simulink model "img_processing"  (R2019b)
settings: Solver=VariableStepAuto  StartTime=0.0  StopTime=10.0  RelTol=1e-3
undefined symbols (not defined in the file or in its folder): none
libraries: imaqlib x1
settings Model: Creator=James  LastModifiedBy=James

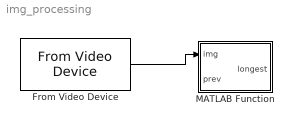
== system img_processing ==
  From Video Device : imaqlib/From Video Device  DeviceMenu=(none)  Device=(none)  ObjConstructor=(none)  VideoFormatMenu=(none)  VideoFormat=(none)  VideoSource=none  ROIPosition=(none)  EnableHWTrigger=off  TriggerConfiguration=none/none  SampleTime=1/30  OutputPortsMode=One multidimensional signal  DataType=single  CanDoHWTrigger=no  ReturnedColorSpace=rgb  BlockHandle=4274.0001  ROIWidth=100  ROIHeight=100  ROIColumn=0  ROIRow=0  EngXMLPath=C:\Program Files\MATLAB\R2019b\toolbox\imaq\imaq\private  DevXMLPath=DEVPATH  EngLibPath=C:\Program Files\MATLAB\R2019b\toolbox\imaq\imaqblks\imaqmex\win64  ColorSpace=rgb  BayerSensorAlignment=grbg  ImaqMode=off
      settings: SourceProductName=Image Acquisition Toolbox
  MATLAB Function : MATLAB Function  TreatAsAtomicUnit=on
  wires:
  From Video Device/1 -> MATLAB Function/1(img)

== matlab function img_processing/MATLAB Function ==
  data: img input; longest output; prev input
function longest  = fcn(img, prev)

    if ~exist('prev', 'var')
        prev1 = [[0,0], [0,0], 400, 0];
        prev2 = [[0,0], [0,0], 400, 0];
        
    else
        prev1 = prev(1);
        prev2 = prev(2);
    end
    
    th_prev = (prev1(3)+prev2(3))/2;
    
    r = img(:,:,1);
    g = img(:,:,2);
    b = img(:,:,3);
    
    justblue = 10*(g-r);
    
    justblue = (justblue > 100);
    ublu = uint8(100*justblue);
    justblue = imgaussfilt(ublu,2);
    
    lines = pipeHough(justblue);
    
    max_len = 0;
    max_len2 = 0;
    max_rho = 0;
    xy_long = [0,0,0,0];
    
    for k = 1:length(lines)
        xy = [lines(k).point1 lines(k).point2];
        th = lines(k).theta;
        rho = lines(k).rho;
        len = norm(lines(k).point1 - lines(k).point2);
        
        p1x = lines(k).point1(1);
        p1y = lines(k).point1(2);
        p2x = lines(k).point2(1);
        p2y = lines(k).point2(2);
        p3x = xy_long(1);
        p3y = xy_long(2);
        p4x = xy_long(3);
        p4y = xy_long(4);
        
        
        A = [p1x - p3x, p2x - p3x; p1y - p3y p2y - p3y];
        B = [p1x-p4x, p2x-p4x; p1y-p4y, p2y-p4y];
        C = [p3x-p1x, p4x-p1x; p3y-p1y, p4y-p1y];
        D = [p3x-p2x, p4x-p2x; p3y-p2y, p4y-p2y];
        
        if (det(A)*det(B) < 0 || det(C)*det(D) < 0)
            inter= true;
        else
            inter = false;
        end

        
       if (len > max_len && (theta_prev == 400 ||abs(th-theta_prev) < 30)&& 20 < abs(rho - max_rho)&& inter == false)
            max_len2 = max_len;
            max_len = len;
            xy_long = lines(k);
            max_rho = rho;
        end
        if (len > max_len2 && (theta_prev == 400 ||abs(th-theta_prev) < 30)&& 20 < abs(rho - max_rho)&& inter == false)
            max_len2 = len;
            xy_long2 = lines(k);
        end
    end
    
    longest = [xy_long xy_long2]

end
